simulink library "VIS_LIB"  (Simulink 8.6)
settings: Solver=ode45  StartTime=0.0  StopTime=10.0  RelTol=1e-3
undefined symbols (not defined in the file): AC, SIXOSEM_F_WD_AC_MASTER
libraries: cdsFilt x376, cdsEpicsOut x253, cdsEpicsIn x179, cdsTP x123, VIS_LIB x95, cdsMuxMatrix x91, cdsEpicsStringIn x75, cdsFiltCtrl x72, cdsFunctionCall x70, cdsRms x59, KAGRA_UTIL x25, STATE_BIO_MASTER x5
(part 8 of 38)

== system VIS_LIB/CrypParts/ADD ==
  ISC_L_In : Inport
  ISC_P_In : Inport  Port=2
  ISC_Y_In : Inport  Port=3
  TEST_L_In : Inport  Port=4
  TEST_P_In : Inport  Port=5
  TEST_Y_In : Inport  Port=6
  Ground{1..6} (6 alike) : Ground
  L : cdsFiltCtrl/IIR FM with control  Tag=cdsFiltCtrl  Description=|
      | cdsFiltCntrl is the standard IIR filter module (exactly the same as cdsFilt) but with added control data output 'Ctrl'. Filter module digital signal output appears on the first output, which is called 'Val'. 'Ctrl' output has a bit pattern encoding the state of filter's on/off switches (FM1 through FM10). The bit values are:
      |                                                                                                                                                                                                                                                                                                                                       
      | module 	hex	dec                                                                                                                                                                                                                                                                                                                       
      | -----------------------                                                                                                                                                                                                                                                                                                               
      | FM1	0x20                    32                                                                                                                                                                                                                                                                                                        
      | FM2	0x80                     128                                                                                                                                                                                                                                                                                                      
      | FM3	0x200                   512                                                                                                                                                                                                                                                                                                       
      | FM4	0x800                   2048                                                                                                                                                                                                                                                                                                      
      | FM5	0x2000                 8192                                                                                                                                                                                                                                                                                                       
      | FM6	0x8000                 32768                                                                                                                                                                                                                                                                                                      
      | FM7	0x20000                131072                                                                                                                                                                                                                                                                                                     
      | FM8	0x80000                 524288                                                                                                                                                                                                                                                                                                    
      | FM9	0x200000               2097152                                                                                                                                                                                                                                                                                                    
      | FM10	0x800000               8388608                                                                                                                                                                                                                                                                                                   
      |                                                                                                                                                                                                                                                                                                                                       
      | This bit data can be used to drive some other switches or it can be output using a binary I/O module.
      settings: AttributesFormatString=%<Tag>
  P : cdsFiltCtrl/IIR FM with control  Tag=cdsFiltCtrl  Description=|
      | cdsFiltCntrl is the standard IIR filter module (exactly the same as cdsFilt) but with added control data output 'Ctrl'. Filter module digital signal output appears on the first output, which is called 'Val'. 'Ctrl' output has a bit pattern encoding the state of filter's on/off switches (FM1 through FM10). The bit values are:
      |                                                                                                                                                                                                                                                                                                                                       
      | module 	hex	dec                                                                                                                                                                                                                                                                                                                       
      | -----------------------                                                                                                                                                                                                                                                                                                               
      | FM1	0x20                    32                                                                                                                                                                                                                                                                                                        
      | FM2	0x80                     128                                                                                                                                                                                                                                                                                                      
      | FM3	0x200                   512                                                                                                                                                                                                                                                                                                       
      | FM4	0x800                   2048                                                                                                                                                                                                                                                                                                      
      | FM5	0x2000                 8192                                                                                                                                                                                                                                                                                                       
      | FM6	0x8000                 32768                                                                                                                                                                                                                                                                                                      
      | FM7	0x20000                131072                                                                                                                                                                                                                                                                                                     
      | FM8	0x80000                 524288                                                                                                                                                                                                                                                                                                    
      | FM9	0x200000               2097152                                                                                                                                                                                                                                                                                                    
      | FM10	0x800000               8388608                                                                                                                                                                                                                                                                                                   
      |                                                                                                                                                                                                                                                                                                                                       
      | This bit data can be used to drive some other switches or it can be output using a binary I/O module.
      settings: AttributesFormatString=%<Tag>
  Sum : Sum
  Sum3 : Sum
  Sum4 : Sum
  Terminator1 : Terminator
  Terminator2 : Terminator
  Terminator3 : Terminator
  Y : cdsFiltCtrl/IIR FM with control  Tag=cdsFiltCtrl  Description=|
      | cdsFiltCntrl is the standard IIR filter module (exactly the same as cdsFilt) but with added control data output 'Ctrl'. Filter module digital signal output appears on the first output, which is called 'Val'. 'Ctrl' output has a bit pattern encoding the state of filter's on/off switches (FM1 through FM10). The bit values are:
      |                                                                                                                                                                                                                                                                                                                                       
      | module 	hex	dec                                                                                                                                                                                                                                                                                                                       
      | -----------------------                                                                                                                                                                                                                                                                                                               
      | FM1	0x20                    32                                                                                                                                                                                                                                                                                                        
      | FM2	0x80                     128                                                                                                                                                                                                                                                                                                      
      | FM3	0x200                   512                                                                                                                                                                                                                                                                                                       
      | FM4	0x800                   2048                                                                                                                                                                                                                                                                                                      
      | FM5	0x2000                 8192                                                                                                                                                                                                                                                                                                       
      | FM6	0x8000                 32768                                                                                                                                                                                                                                                                                                      
      | FM7	0x20000                131072                                                                                                                                                                                                                                                                                                     
      | FM8	0x80000                 524288                                                                                                                                                                                                                                                                                                    
      | FM9	0x200000               2097152                                                                                                                                                                                                                                                                                                    
      | FM10	0x800000               8388608                                                                                                                                                                                                                                                                                                   
      |                                                                                                                                                                                                                                                                                                                                       
      | This bit data can be used to drive some other switches or it can be output using a binary I/O module.
      settings: AttributesFormatString=%<Tag>
  LONG_Out : Outport
  PITCH_Out : Outport  Port=2
  YAW_Out : Outport  Port=3
  wires:
  ISC_L_In/1 -> Sum/1
  TEST_L_In/1 -> Sum/2
  ISC_Y_In/1 -> Sum3/1
  TEST_Y_In/1 -> Sum3/2
  TEST_P_In/1 -> Sum4/2
  ISC_P_In/1 -> Sum4/1
  Sum/1 -> L/1
  Ground1/1 -> L/3
  Ground6/1 -> L/2
  L/1 -> LONG_Out/1
  Sum4/1 -> P/1
  Ground2/1 -> P/3
  Ground3/1 -> P/2
  P/1 -> PITCH_Out/1
  Sum3/1 -> Y/1
  Ground4/1 -> Y/3
  Ground5/1 -> Y/2
  Y/1 -> YAW_Out/1
  L/2 -> Terminator1/1
  P/2 -> Terminator2/1
  Y/2 -> Terminator3/1

== system VIS_LIB/CrypParts/ADDALL ==
  ISC_L_In : Inport
  ISC_P_In : Inport  Port=2
  ISC_Y_In : Inport  Port=3
  LOCAL_L_In : Inport  Port=4
  LOCAL_T_In : Inport  Port=5
  LOCAL_V_In : Inport  Port=6
  LOCAL_R_In : Inport  Port=7
  LOCAL_P_In : Inport  Port=8
  LOCAL_Y_In : Inport  Port=9
  Sum1 : Sum
  Sum2 : Sum
  Sum3 : Sum  Inputs=+
  Sum4 : Sum  Inputs=+
  Sum5 : Sum
  Sum6 : Sum  Inputs=+
  LONG_MAIN_Out : Outport
  TRANS_MAIN_Out : Outport  Port=2
  VERT_MAIN_Out : Outport  Port=3
  ROLL_MAIN_Out : Outport  Port=4
  PITCH_MAIN_Out : Outport  Port=5
  YAW_MAIN_Out : Outport  Port=6
  wires:
  ISC_L_In/1 -> [ISC_L]
  ISC_P_In/1 -> [ISC_P]
  ISC_Y_In/1 -> [ISC_Y]
  LOCAL_L_In/1 -> [DAMP_L]
  LOCAL_P_In/1 -> [DAMP_P]
  LOCAL_Y_In/1 -> [DAMP_Y]
  [DAMP_L] -> Sum1/2
  [ISC_L] -> Sum1/1
  Sum5/1 -> PITCH_MAIN_Out/1
  Sum1/1 -> LONG_MAIN_Out/1
  [ISC_Y] -> Sum2/1
  [DAMP_Y] -> Sum2/2
  Sum2/1 -> YAW_MAIN_Out/1
  [ISC_P] -> Sum5/1
  [DAMP_P] -> Sum5/2
  LOCAL_T_In/1 -> Sum3/1
  Sum3/1 -> TRANS_MAIN_Out/1
  LOCAL_V_In/1 -> Sum4/1
  Sum4/1 -> VERT_MAIN_Out/1
  LOCAL_R_In/1 -> Sum6/1
  Sum6/1 -> ROLL_MAIN_Out/1

== system VIS_LIB/CrypParts/ADDISC_IM ==
  LOCK_L_In : Inport
  LOCK_P_In : Inport  Port=2
  LOCK_Y_In : Inport  Port=3
  DITHER_P_In : Inport  Port=4
  DITHER_Y_In : Inport  Port=5
  CALLINE_L_In : Inport  Port=6
  Sum1 : Sum
  Sum3 : Sum
  Sum4 : Sum
  LONG_ISC_Out : Outport
  PITCH_ISC_Out : Outport  Port=2
  YAW_ISC_Out : Outport  Port=3
  wires:
  Sum3/1 -> YAW_ISC_Out/1
  Sum4/1 -> PITCH_ISC_Out/1
  DITHER_P_In/1 -> [DITHER_P]
  DITHER_Y_In/1 -> [DITHER_Y]
  LOCK_P_In/1 -> [LOCK_P]
  LOCK_Y_In/1 -> [LOCK_Y]
  [DITHER_P] -> Sum4/2
  [LOCK_P] -> Sum4/1
  [LOCK_Y] -> Sum3/1
  [DITHER_Y] -> Sum3/2
  LOCK_L_In/1 -> Sum1/1
  Sum1/1 -> LONG_ISC_Out/1
  CALLINE_L_In/1 -> [CALLINE_L]
  [CALLINE_L] -> Sum1/2

== system VIS_LIB/CrypParts/ADDISC_MN ==
  LOCK_L_In : Inport
  LOCK_P_In : Inport  Port=2
  LOCK_Y_In : Inport  Port=3
  DITHER_P_In : Inport  Port=4
  DITHER_Y_In : Inport  Port=5
  OPTICALIGN_P_In : Inport  Port=6
  OPTICALIGN_Y_In : Inport  Port=7
  CALLINE_L_In : Inport  Port=8
  Sum1 : Sum
  Sum3 : Sum  Inputs=+++
  Sum4 : Sum  Inputs=+++
  LONG_ISC_Out : Outport
  PITCH_ISC_Out : Outport  Port=2
  YAW_ISC_Out : Outport  Port=3
  wires:
  Sum3/1 -> YAW_ISC_Out/1
  Sum4/1 -> PITCH_ISC_Out/1
  OPTICALIGN_P_In/1 -> [OPTICALIGN_P]
  OPTICALIGN_Y_In/1 -> [OPTICALIGN_Y]
  DITHER_P_In/1 -> [DITHER_P]
  DITHER_Y_In/1 -> [DITHER_Y]
  LOCK_P_In/1 -> [LOCK_P]
  LOCK_Y_In/1 -> [LOCK_Y]
  [DITHER_P] -> Sum4/2
  [LOCK_P] -> Sum4/1
  [OPTICALIGN_P] -> Sum4/3
  [OPTICALIGN_Y] -> Sum3/3
  [LOCK_Y] -> Sum3/1
  [DITHER_Y] -> Sum3/2
  LOCK_L_In/1 -> Sum1/1
  Sum1/1 -> LONG_ISC_Out/1
  CALLINE_L_In/1 -> [CALLINE_L]
  [CALLINE_L] -> Sum1/2

== system VIS_LIB/CrypParts/ADDLOCAL_IM ==
  note: Sending OLSERVO signals with Goto/From blocks will spoil the make process.
      | Error message: "Please check the model for missing links around these parts."
      | --- K.Okutomi, June 2019
  TEST_L_In : Inport
  TEST_T_In : Inport  Port=2
  TEST_V_In : Inport  Port=3
  TEST_R_In : Inport  Port=4
  TEST_P_In : Inport  Port=5
  TEST_Y_In : Inport  Port=6
  PSDAMP_L_In : Inport  Port=7
  PSDAMP_T_In : Inport  Port=8
  PSDAMP_V_In : Inport  Port=9
  PSDAMP_R_In : Inport  Port=10
  PSDAMP_P_In : Inport  Port=11
  PSDAMP_Y_In : Inport  Port=12
  TMOLDAMP_L_In : Inport  Port=13
  TMOLDAMP_P_In : Inport  Port=14
  TMOLDAMP_Y_In : Inport  Port=15
  OLSERVO_L_In : Inport  Port=16
  OLSERVO_T_In : Inport  Port=17
  OLSERVO_V_In : Inport  Port=18
  OLSERVO_R_In : Inport  Port=19
  OLSERVO_P_In : Inport  Port=20
  OLSERVO_Y_In : Inport  Port=21
  Sum : Sum  Inputs=++++
  Sum1 : Sum  Inputs=+++
  Sum2 : Sum  Inputs=+++
  Sum3 : Sum  Inputs=++++
  Sum4 : Sum  Inputs=++++
  Sum5 : Sum  Inputs=+++
  LONG_LOCAL_Out : Outport
  TRANS_LOCAL_Out : Outport  Port=2
  VERT_LOCAL_Out : Outport  Port=3
  ROLL_LOCAL_Out : Outport  Port=4
  PITCH_LOCAL_Out : Outport  Port=5
  YAW_LOCAL_Out : Outport  Port=6
  wires:
  [PSDAMP_Y] -> Sum3/2
  [PSDAMP_P] -> Sum4/2
  [TEST_Y] -> Sum3/1
  [TEST_P] -> Sum4/1
  [PSDAMP_R] -> Sum5/2
  [PSDAMP_V] -> Sum2/2
  [TEST_R] -> Sum5/1
  [TEST_V] -> Sum2/1
  [PSDAMP_T] -> Sum1/2
  [TEST_T] -> Sum1/1
  [TMOLDAMP_L] -> Sum/3
  [PSDAMP_L] -> Sum/2
  TEST_Y_In/1 -> [TEST_Y]
  TEST_P_In/1 -> [TEST_P]
  TEST_R_In/1 -> [TEST_R]
  TEST_V_In/1 -> [TEST_V]
  TEST_T_In/1 -> [TEST_T]
  TEST_L_In/1 -> [TEST_L]
  PSDAMP_Y_In/1 -> [PSDAMP_Y]
  PSDAMP_P_In/1 -> [PSDAMP_P]
  PSDAMP_R_In/1 -> [PSDAMP_R]
  PSDAMP_V_In/1 -> [PSDAMP_V]
  PSDAMP_T_In/1 -> [PSDAMP_T]
  PSDAMP_L_In/1 -> [PSDAMP_L]
  [TEST_L] -> Sum/1
  TMOLDAMP_Y_In/1 -> [TMOLDAMP_Y]
  TMOLDAMP_P_In/1 -> [TMOLDAMP_P]
  TMOLDAMP_L_In/1 -> [TMOLDAMP_L]
  Sum1/1 -> TRANS_LOCAL_Out/1
  Sum2/1 -> VERT_LOCAL_Out/1
  Sum5/1 -> ROLL_LOCAL_Out/1
  Sum/1 -> LONG_LOCAL_Out/1
  Sum3/1 -> YAW_LOCAL_Out/1
  Sum4/1 -> PITCH_LOCAL_Out/1
  [TMOLDAMP_Y] -> Sum3/3
  [TMOLDAMP_P] -> Sum4/3
  OLSERVO_L_In/1 -> [OLSERVO_L]
  OLSERVO_T_In/1 -> [OLSERVO_T]
  OLSERVO_V_In/1 -> [OLSERVO_V]
  OLSERVO_R_In/1 -> [OLSERVO_R]
  OLSERVO_P_In/1 -> [OLSERVO_P]
  OLSERVO_Y_In/1 -> [OLSERVO_Y]
  [OLSERVO_L] -> Sum/4
  [OLSERVO_T] -> Sum1/3
  [OLSERVO_V] -> Sum2/3
  [OLSERVO_R] -> Sum5/3
  [OLSERVO_P] -> Sum4/4
  [OLSERVO_Y] -> Sum3/4

== system VIS_LIB/CrypParts/ADDLOCAL_MN ==
  note: Sending OLSERVO signals with Goto/From blocks will spoil the make process.
      | Error message: "Please check the model for missing links around these parts."
      | --- K.Okutomi, June 2019
  TEST_L_In : Inport
  TEST_T_In : Inport  Port=2
  TEST_V_In : Inport  Port=3
  TEST_R_In : Inport  Port=4
  TEST_P_In : Inport  Port=5
  TEST_Y_In : Inport  Port=6
  PSDAMP_L_In : Inport  Port=7
  PSDAMP_T_In : Inport  Port=8
  PSDAMP_V_In : Inport  Port=9
  PSDAMP_R_In : Inport  Port=10
  PSDAMP_P_In : Inport  Port=11
  PSDAMP_Y_In : Inport  Port=12
  MNOLDAMP_P_In : Inport  Port=13
  MNOLDAMP_Y_In : Inport  Port=14
  TMOLDAMP_L_In : Inport  Port=15
  TMOLDAMP_P_In : Inport  Port=16
  TMOLDAMP_Y_In : Inport  Port=17
  OLSERVO_L_In : Inport  Port=18
  OLSERVO_T_In : Inport  Port=19
  OLSERVO_V_In : Inport  Port=20
  OLSERVO_R_In : Inport  Port=21
  OLSERVO_P_In : Inport  Port=22
  OLSERVO_Y_In : Inport  Port=23
  OLDCCTRL_P_In : Inport  Port=24
  OLDCCTRL_Y_In : Inport  Port=25
  Sum : Sum  Inputs=++++
  Sum1 : Sum  Inputs=+++
  Sum2 : Sum  Inputs=+++
  Sum3 : Sum  Inputs=++++++
  Sum4 : Sum  Inputs=++++++
  Sum5 : Sum  Inputs=+++
  LONG_LOCAL_Out : Outport
  TRANS_LOCAL_Out : Outport  Port=2
  VERT_LOCAL_Out : Outport  Port=3
  ROLL_LOCAL_Out : Outport  Port=4
  PITCH_LOCAL_Out : Outport  Port=5
  YAW_LOCAL_Out : Outport  Port=6
  wires:
  [TMOLDAMP_Y] -> Sum3/4
  [TMOLDAMP_P] -> Sum4/4
  [MNOLDAMP_P] -> Sum4/3
  [MNOLDAMP_Y] -> Sum3/3
  [PSDAMP_Y] -> Sum3/2
  [PSDAMP_P] -> Sum4/2
  [TEST_Y] -> Sum3/1
  [TEST_P] -> Sum4/1
  [PSDAMP_R] -> Sum5/2
  [PSDAMP_V] -> Sum2/2
  [TEST_R] -> Sum5/1
  [TEST_V] -> Sum2/1
  [PSDAMP_T] -> Sum1/2
  [TEST_T] -> Sum1/1
  [TMOLDAMP_L] -> Sum/3
  [PSDAMP_L] -> Sum/2
  MNOLDAMP_Y_In/1 -> [MNOLDAMP_Y]
  MNOLDAMP_P_In/1 -> [MNOLDAMP_P]
  TEST_Y_In/1 -> [TEST_Y]
  TEST_P_In/1 -> [TEST_P]
  TEST_R_In/1 -> [TEST_R]
  TEST_V_In/1 -> [TEST_V]
  TEST_T_In/1 -> [TEST_T]
  TEST_L_In/1 -> [TEST_L]
  PSDAMP_Y_In/1 -> [PSDAMP_Y]
  PSDAMP_P_In/1 -> [PSDAMP_P]
  PSDAMP_R_In/1 -> [PSDAMP_R]
  PSDAMP_V_In/1 -> [PSDAMP_V]
  PSDAMP_T_In/1 -> [PSDAMP_T]
  PSDAMP_L_In/1 -> [PSDAMP_L]
  [TEST_L] -> Sum/1
  TMOLDAMP_Y_In/1 -> [TMOLDAMP_Y]
  TMOLDAMP_P_In/1 -> [TMOLDAMP_P]
  TMOLDAMP_L_In/1 -> [TMOLDAMP_L]
  Sum1/1 -> TRANS_LOCAL_Out/1
  Sum2/1 -> VERT_LOCAL_Out/1
  Sum5/1 -> ROLL_LOCAL_Out/1
  Sum/1 -> LONG_LOCAL_Out/1
  Sum3/1 -> YAW_LOCAL_Out/1
  Sum4/1 -> PITCH_LOCAL_Out/1
  OLSERVO_L_In/1 -> [OLSERVO_L]
  [OLSERVO_L] -> Sum/4
  OLSERVO_T_In/1 -> [OLSERVO_T]
  OLSERVO_V_In/1 -> [OLSERVO_V]
  OLSERVO_R_In/1 -> [OLSERVO_R]
  OLSERVO_P_In/1 -> [OLSERVO_P]
  OLSERVO_Y_In/1 -> [OLSERVO_Y]
  [OLSERVO_T] -> Sum1/3
  [OLSERVO_V] -> Sum2/3
  [OLSERVO_R] -> Sum5/3
  [OLSERVO_P] -> Sum4/5
  [OLSERVO_Y] -> Sum3/5
  OLDCCTRL_Y_In/1 -> [OLDCCTRL_Y]
  OLDCCTRL_P_In/1 -> [OLDCCTRL_P]
  [OLDCCTRL_P] -> Sum4/6
  [OLDCCTRL_Y] -> Sum3/6

== system VIS_LIB/CrypParts/ADD_TM ==
  LOCK_L_In : Inport
  LOCK_P_In : Inport  Port=2
  LOCK_Y_In : Inport  Port=3
  DITHER_P_In : Inport  Port=4
  DITHER_Y_In : Inport  Port=5
  TEST_L_In : Inport  Port=6
  TEST_P_In : Inport  Port=7
  TEST_Y_In : Inport  Port=8
  DAMP_L_In : Inport  Port=9
  DAMP_P_In : Inport  Port=10
  DAMP_Y_In : Inport  Port=11
  OLSERVO_L_In : Inport  Port=12
  OLSERVO_P_In : Inport  Port=13
  OLSERVO_Y_In : Inport  Port=14
  CALLINE_L_In : Inport  Port=15
  Sum1 : Sum  Inputs=+++++
  Sum2 : Sum  Inputs=+++++
  Sum5 : Sum  Inputs=+++++
  LONG_MAIN_Out : Outport
  PITCH_MAIN_Out : Outport  Port=2
  YAW_MAIN_Out : Outport  Port=3
  wires:
  LOCK_L_In/1 -> [ISC_L]
  LOCK_P_In/1 -> [ISC_P]
  LOCK_Y_In/1 -> [ISC_Y]
  DAMP_L_In/1 -> [DAMP_L]
  DAMP_P_In/1 -> [DAMP_P]
  DAMP_Y_In/1 -> [DAMP_Y]
  [ISC_L] -> Sum1/1
  Sum5/1 -> PITCH_MAIN_Out/1
  Sum1/1 -> LONG_MAIN_Out/1
  [ISC_Y] -> Sum2/1
  Sum2/1 -> YAW_MAIN_Out/1
  [ISC_P] -> Sum5/1
  TEST_Y_In/1 -> [TEST_Y]
  TEST_P_In/1 -> [TEST_P]
  TEST_L_In/1 -> [TEST_L]
  DITHER_P_In/1 -> [DITHER_P]
  DITHER_Y_In/1 -> [DITHER_Y]
  [DAMP_Y] -> Sum2/4
  [DITHER_Y] -> Sum2/2
  [TEST_Y] -> Sum2/3
  [DAMP_P] -> Sum5/4
  [TEST_P] -> Sum5/3
  [DITHER_P] -> Sum5/2
  [DAMP_L] -> Sum1/3
  [TEST_L] -> Sum1/2
  OLSERVO_L_In/1 -> [OLSERVO_L]
  OLSERVO_P_In/1 -> [OLSERVO_P]
  OLSERVO_Y_In/1 -> [OLSERVO_Y]
  [OLSERVO_L] -> Sum1/4
  [OLSERVO_P] -> Sum5/5
  [OLSERVO_Y] -> Sum2/5
  CALLINE_L_In/1 -> [CALLINE_L]
  [CALLINE_L] -> Sum1/5
